simulink subsystem "BaseballAero"  (R2024b)
settings: Solver=VariableStepAuto  StartTime=0.0  StopTime=10.0  RelTol=1e-3
undefined symbols (not defined in the file): SimIn
settings Model: Creator=macheson  LastModifiedBy=macheson

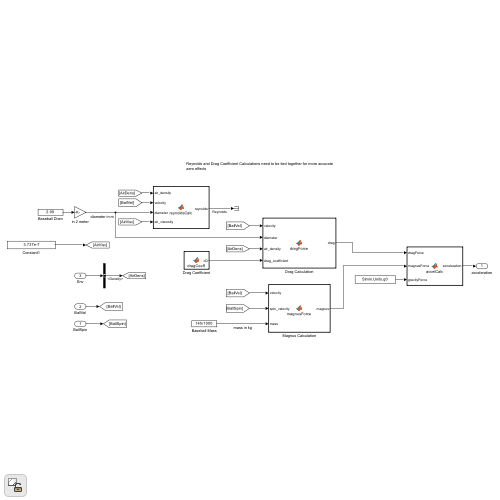
[thumbnail: Simulink's stored preview of the top-level diagram]
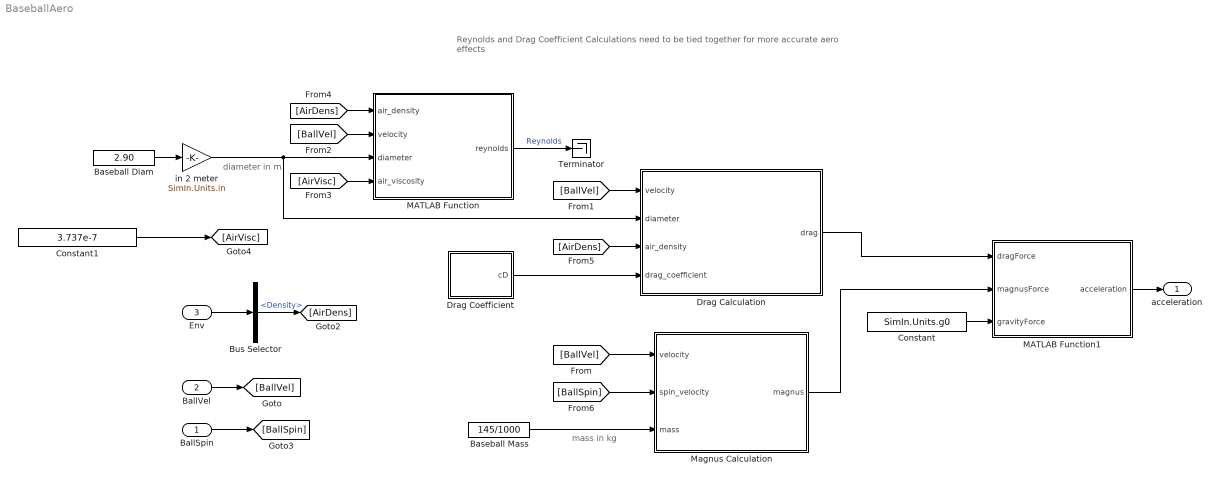
== system BaseballAero ==
  note: mass in kg
  note: Reynolds and Drag Coefficient Calculations need to be tied together for more accurate aero effects
  note: diameter in m
  BallSpin : Inport
  BallVel : Inport  Port=2
  Env : Inport  Port=3
  Baseball Diam : Constant  Value=2.90
  Baseball Mass : Constant  Value=145/1000
  Bus Selector : BusSelector  OutputSignals=Atmosphere.Density
  Constant : Constant  Value=SimIn.Units.g0
  Constant1 : Constant  Value=3.737e-7  VectorParams1D=off  SampleTime=-1
  Drag Calculation : MATLAB Function  TreatAsAtomicUnit=on
  Drag Coefficient : MATLAB Function  TreatAsAtomicUnit=on
  MATLAB Function : MATLAB Function  TreatAsAtomicUnit=on
  MATLAB Function1 : MATLAB Function  TreatAsAtomicUnit=on
  Magnus Calculation : MATLAB Function  TreatAsAtomicUnit=on
  Terminator : Terminator
  in 2 meter : Gain  Gain=SimIn.Units.in
  acceleration : Outport
  wires:
  Drag Coefficient/1(cD) -> Drag Calculation/4(drag_coefficient)
  Constant/1 -> MATLAB Function1/3(gravityForce)
  MATLAB Function/1(reynolds) -> Terminator/1  "Reynolds"
  Magnus Calculation/1(magnus) -> MATLAB Function1/2(magnusForce)
  Baseball Diam/1 -> in 2 meter/1
  Drag Calculation/1(drag) -> MATLAB Function1/1(dragForce)
  MATLAB Function1/1(acceleration) -> acceleration/1
  Baseball Mass/1 -> Magnus Calculation/3(mass)
  BallSpin/1 -> [BallSpin]
  Env/1 -> Bus Selector/1
  BallVel/1 -> [BallVel]
  [BallVel] -> Magnus Calculation/1(velocity)
  [BallVel] -> Drag Calculation/1(velocity)
  [BallVel] -> MATLAB Function/2(velocity)
  [AirVisc] -> MATLAB Function/4(air_viscosity)
  Bus Selector/1 -> [AirDens]  "<Density>"
  [AirDens] -> MATLAB Function/1(air_density)
  [AirDens] -> Drag Calculation/3(air_density)
  [BallSpin] -> Magnus Calculation/2(spin_velocity)
  in 2 meter/1 -> Drag Calculation/2(diameter), MATLAB Function/3(diameter)
  Constant1/1 -> [AirVisc]

== matlab function BaseballAero/Drag Calculation ==
  data: velocity input; drag output; diameter input; air_density input; drag_coefficient input
function drag = dragForce(velocity, diameter, air_density, drag_coefficient)

area = pi*(diameter.^2)./4;

%drag = 0.5*area*drag_coefficient*air_density.*abs(velocity).*velocity;

drag = -1*(0.0039 + 0.0058/(1 + exp((norm(velocity) - 35)/5)))*norm(velocity);


end

== matlab function BaseballAero/Drag Coefficient ==
  data: cD output
function cD = dragCoeff()

cD = 0.3;

== matlab function BaseballAero/MATLAB Function ==
  data: air_density input; reynolds output; velocity input; diameter input; air_viscosity input
function reynolds = reynoldsCalc(air_density, velocity, diameter, air_viscosity)
reynolds = air_density*norm(velocity)*diameter/air_viscosity;

== matlab function BaseballAero/MATLAB Function1 ==
  data: dragForce input; acceleration output; magnusForce input; gravityForce input
function acceleration = accelCalc(dragForce, magnusForce, gravityForce)

acceleration = magnusForce - dragForce + gravityForce;

end

== matlab function BaseballAero/Magnus Calculation ==
  data: magnus output; velocity input; spin_velocity input; mass input
function magnus = magnusForce(velocity, spin_velocity, mass)

magnus = magnusForce(velocity, spin_velocity, mass);

end
